simulink model "SetBelt"  (R2024a)
settings: Solver=FixedStepAuto  StartTime=0.0  StopTime=30  RelTol=1e-3
undefined symbols (not defined in the file): Dem_EventStatusType, enState_IgnitionKey
libraries: simulink x7, autosarlibnvm x3, autosarlibdem x2, dspswit3 x1
settings Model: Creator=buiqu  LastModifiedBy=buiqu
settings OptimizationCC: DefaultParameterBehavior=Inlined  EnhancedBackFolding=on  PassReuseOutputArgsAs=Individual arguments  ZeroExternalMemoryAtStartup=off  ZeroInternalMemoryAtStartup=off  OptimizeBlockOrder=speed  DifferentSizesBufferReuse=on  OptimizationCustomize=off  EfficientTunableParamExpr=on
settings DebuggingCC: ParameterTunabilityLossMsg=error
settings SFSimCC: MATLABDynamicMemAlloc=off
settings RTWCC: Description=AUTOSAR  SystemTargetFile=autosar.tlc  GenCodeOnly=on  TemplateMakefile=ert_default_tmf  DataTypeReplacement=CDataTypesFixedWidth
settings CodeAppCC: ForceParamTrailComments=on  IgnoreCustomStorageClasses=off  OperatorAnnotations=on  SimulinkDataObjDesc=on  SFDataObjDesc=on  InsertBlockDesc=on
settings STFCustomTargetCC: MultiwordLength=256  ParMdlRefBuildCompliant=on  CompOptLevelCompliant=on  CombineOutputUpdateFcns=on  SuppressErrorStatus=on  ERTCustomFileBanners=on  SupportNonFinite=off  SupportComplex=off  SupportContinuousTime=off  SupportNonInlinedSFcns=off  RemoveResetFunc=on  MATLABClassNameForMDSCustomization=Simulink.SoftwareTarget.ERTCustomization  AutosarCompliant=on  GRTInterface=off  LookupTableObjectStructAxisOrder=2,1,3,4,...  LUTObjectStructOrderEvenSpacing=Size,Table,Breakpoints  SystemTargetFile=autosar.tlc
settings ERTTargetCC: TargetLangStandard=C99 (ISO)  ConcurrentExecutionCompliant=off  SuppressErrorStatus=on  SupportNonFinite=off  SupportComplex=off  ModelStepFunctionPrototypeControlCompliant=off  CPPClassGenCompliant=off  AutosarCompliant=on  LookupTableObjectStructAxisOrder=2,1,3,4,...  LUTObjectStructOrderEvenSpacing=Size,Table,Breakpoints  InlinedParameterPlacement=NonHierarchical  ERTCustomFileTemplate=example_file_process.tlc  BooleanTrueId=TRUE  BooleanFalseId=FALSE

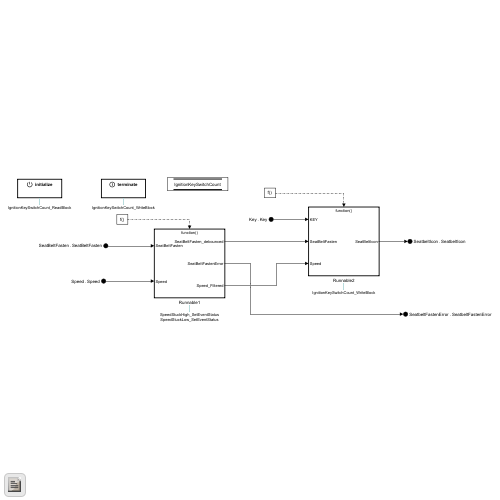
[thumbnail: Simulink's stored preview of the top-level diagram]
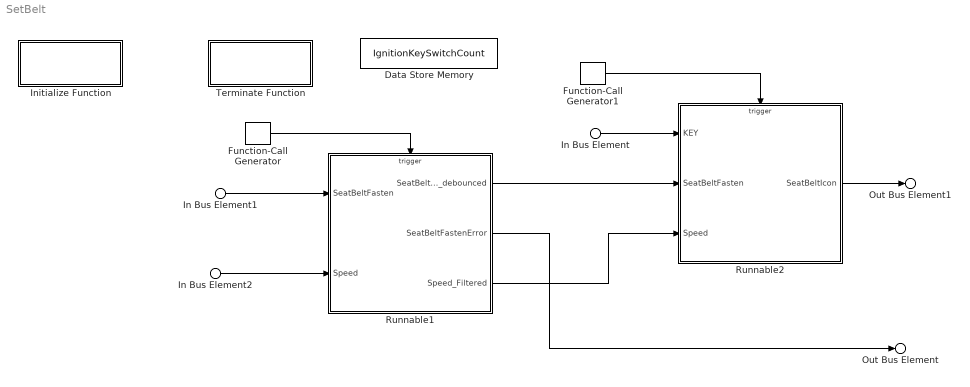
== system SetBelt ==
  In Bus Element : Inport  PortName=Key  Element=Key
  In Bus Element1 : Inport  Port=2  PortName=SeatBeltFasten  Element=SeatBeltFasten
  In Bus Element2 : Inport  Port=3  PortName=Speed  Element=Speed
  Data Store Memory : DataStoreMemory  DataStoreName=IgnitionKeySwitchCount  WriteAfterWriteMsg=warning  ShowAdditionalParam=off
  Function-Call Generator : simulink/Ports & Subsystems/Function-Call Generator  sample_time=1  numberOfIterations=1  DisallowWideOutput=off
  Function-Call Generator1 : simulink/Ports & Subsystems/Function-Call Generator  sample_time=1  numberOfIterations=1  DisallowWideOutput=off
  Initialize Function : Subsystem  TreatAsAtomicUnit=on
  Runnable1 : Subsystem  TreatAsAtomicUnit=on
  Runnable2 : Subsystem  TreatAsAtomicUnit=on
  Terminate Function : Subsystem  TreatAsAtomicUnit=on
  Out Bus Element1 : Outport  PortName=SeatbeltIcon  Element=SeatbeltIcon
  Out Bus Element : Outport  Port=2  PortName=SeatbeltFastenError  Element=SeatbeltFastenError
  wires:
  Runnable1/3(Speed_Filtered) -> Runnable2/3(Speed)
  Function-Call Generator/1 -> Runnable1/Trigger
  Runnable1/1(SeatBeltFasten_debounced) -> Runnable2/2(SeatBeltFasten)
  Function-Call Generator1/1 -> Runnable2/Trigger
  In Bus Element/1 -> Runnable2/1(KEY)
  In Bus Element1/1 -> Runnable1/1(SeatBeltFasten)
  In Bus Element2/1 -> Runnable1/2(Speed)
  Runnable1/2(SeatBeltFastenError) -> Out Bus Element/1
  Runnable2/1(SeatBeltIcon) -> Out Bus Element1/1

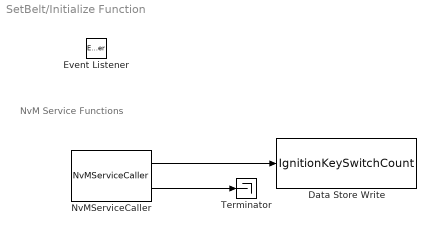
== system SetBelt/Initialize Function ==
  note: NvM Service Functions
  Data Store Write : DataStoreWrite  DataStoreName=IgnitionKeySwitchCount  IndexOptions=Index vector (dialog)  Indices=1  OutputSizes=1
  Event Listener : EventListener  DisableCoverage=on  EventName=reset
  NvMServiceCaller : autosarlibnvm/NvMServiceCaller  PortName=IgnitionKeySwitchCount  Operation=ReadBlock  ArgumentSpecification=uint8(1)  st=-1  ServiceImpl=autosar.bsw.NvMService  SyncToSchema=off
  Terminator : Terminator
  wires:
  NvMServiceCaller/2 -> Terminator/1
  NvMServiceCaller/1 -> Data Store Write/1

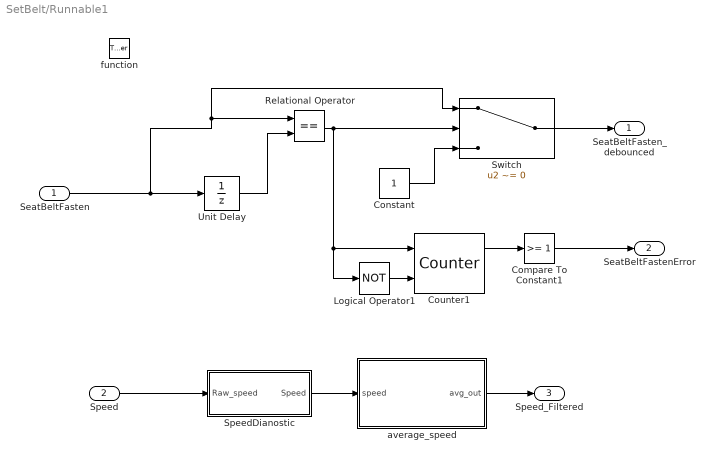
== system SetBelt/Runnable1 ==
  SeatBeltFasten : Inport
  Speed : Inport  Port=2  OutDataTypeStr=uint16
  function : TriggerPort  TriggerType=function-call  VariantControl=(inherit)
  Compare To Constant1 : simulink/Logic and Bit Operations/Compare To Constant  relop=>=  const=1  OutDataTypeStr=boolean
  Constant : Constant
  Counter1 : dspswit3/Counter  Direction=Up  CountEvent=Falling edge  CounterSize=User defined  MaxCount=3  InitialCount=0  Output=Count and Hit  HitValue=1  ResetInput=on  SamplesPerFrame=1  Ts=1  CntDtype=double  HitDtype=Boolean
  Logical Operator1 : Logic  Operator=NOT  AllPortsSameDT=off  OutDataTypeStr=boolean
  Relational Operator : RelationalOperator  Operator===  OutDataTypeStr=boolean  RndMeth=Simplest  InputSameDT=off
  SpeedDianostic : Subsystem
  Switch : Switch  Criteria=u2 ~= 0  OutDataTypeStr=boolean  SaturateOnIntegerOverflow=off  InputSameDT=off
  Unit Delay : UnitDelay  SampleTime=-1  HasFrameUpgradeWarning=on
  average_speed : MATLAB Function  TreatAsAtomicUnit=on
  SeatBeltFasten_debounced : Outport  OutMin=0  OutMax=1  OutDataTypeStr=boolean
  SeatBeltFastenError : Outport  Port=2  OutMin=0  OutMax=1  OutDataTypeStr=boolean
  Speed_Filtered : Outport  Port=3  OutDataTypeStr=uint16
  wires:
  SeatBeltFasten/1 -> Switch/1, Relational Operator/1, Unit Delay/1
  Speed/1 -> SpeedDianostic/1(Raw_speed)
  SpeedDianostic/1(Speed) -> average_speed/1(speed)
  average_speed/1(avg_out) -> Speed_Filtered/1
  Unit Delay/1 -> Relational Operator/2
  Relational Operator/1 -> Logical Operator1/1, Counter1/1, Switch/2
  Switch/1 -> SeatBeltFasten_debounced/1
  Constant/1 -> Switch/3
  Counter1/1 -> Compare To Constant1/1
  Compare To Constant1/1 -> SeatBeltFastenError/1
  Logical Operator1/1 -> Counter1/2

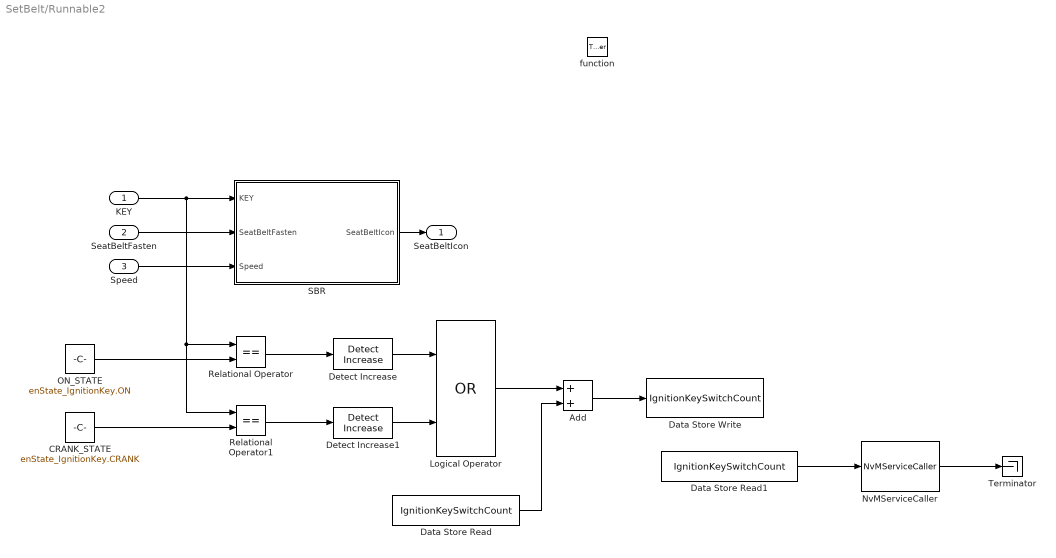
== system SetBelt/Runnable2 ==
  KEY : Inport  OutDataTypeStr=Enum: enState_IgnitionKey
  SeatBeltFasten : Inport  Port=2  OutDataTypeStr=boolean
  Speed : Inport  Port=3  OutDataTypeStr=uint16
  function : TriggerPort  TriggerType=function-call  VariantControl=(inherit)
  Add : Sum
  CRANK_STATE : Constant  Value=enState_IgnitionKey.CRANK  OutDataTypeStr=Enum: enState_IgnitionKey
  Data Store Read : DataStoreRead  DataStoreName=IgnitionKeySwitchCount  IndexOptions=Index vector (dialog)  Indices=1  OutputSizes=1
  Data Store Read1 : DataStoreRead  DataStoreName=IgnitionKeySwitchCount  IndexOptions=Index vector (dialog)  Indices=1  OutputSizes=1
  Data Store Write : DataStoreWrite  DataStoreName=IgnitionKeySwitchCount  IndexOptions=Index vector (dialog)  Indices=1  OutputSizes=1
  Detect Increase : simulink/Logic and Bit Operations/Detect Increase  vinit=0.0  OutDataTypeStr=boolean
  Detect Increase1 : simulink/Logic and Bit Operations/Detect Increase  vinit=0.0  OutDataTypeStr=boolean
  Logical Operator : Logic  Operator=OR  AllPortsSameDT=off  OutDataTypeStr=boolean
  NvMServiceCaller : autosarlibnvm/NvMServiceCaller  PortName=IgnitionKeySwitchCount  Operation=WriteBlock  ArgumentSpecification=uint8(1)  st=-1  ServiceImpl=autosar.bsw.NvMService  SyncToSchema=off
  ON_STATE : Constant  Value=enState_IgnitionKey.ON  OutDataTypeStr=Enum: enState_IgnitionKey
  Relational Operator : RelationalOperator  Operator===  OutDataTypeStr=boolean  RndMeth=Simplest  InputSameDT=off
  Relational Operator1 : RelationalOperator  Operator===  OutDataTypeStr=boolean  RndMeth=Simplest  InputSameDT=off
  SBR : Subsystem
  Terminator : Terminator
  SeatBeltIcon : Outport  OutDataTypeStr=boolean
  wires:
  KEY/1 -> Relational Operator1/1, Relational Operator/1, SBR/1(KEY)
  SeatBeltFasten/1 -> SBR/2(SeatBeltFasten)
  Speed/1 -> SBR/3(Speed)
  ON_STATE/1 -> Relational Operator/2
  CRANK_STATE/1 -> Relational Operator1/2
  Relational Operator/1 -> Detect Increase/1
  Relational Operator1/1 -> Detect Increase1/1
  Detect Increase1/1 -> Logical Operator/2
  Detect Increase/1 -> Logical Operator/1
  Logical Operator/1 -> Add/1
  Data Store Read/1 -> Add/2
  Add/1 -> Data Store Write/1
  Data Store Read1/1 -> NvMServiceCaller/1
  NvMServiceCaller/1 -> Terminator/1
  SBR/1(SeatBeltIcon) -> SeatBeltIcon/1

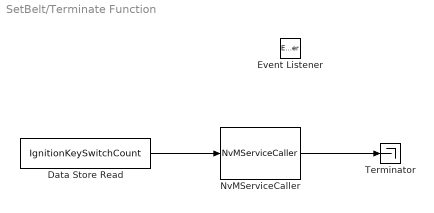
== system SetBelt/Terminate Function ==
  Data Store Read : DataStoreRead  DataStoreName=IgnitionKeySwitchCount  IndexOptions=Index vector (dialog)  Indices=1  OutputSizes=1
  Event Listener : EventListener  DisableCoverage=on  EventType=Terminate  EventName=reset
  NvMServiceCaller : autosarlibnvm/NvMServiceCaller  PortName=IgnitionKeySwitchCount  Operation=WriteBlock  ArgumentSpecification=uint8(1)  st=-1  ServiceImpl=autosar.bsw.NvMService  SyncToSchema=off
  Terminator : Terminator
  wires:
  Data Store Read/1 -> NvMServiceCaller/1
  NvMServiceCaller/1 -> Terminator/1

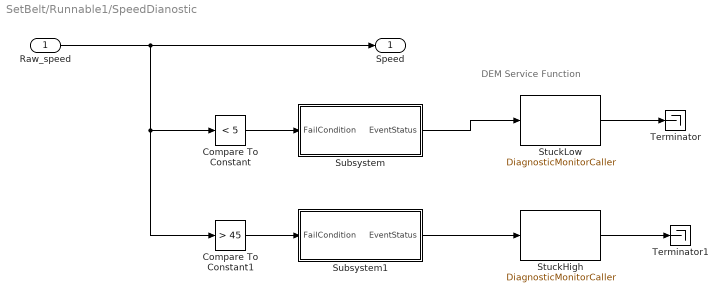
== system SetBelt/Runnable1/SpeedDianostic ==
  note: DEM Service Function
  Raw_speed : Inport  OutDataTypeStr=uint16
  Compare To Constant : simulink/Logic and Bit Operations/Compare To Constant  relop=<  const=5  OutDataTypeStr=boolean
  Compare To Constant1 : simulink/Logic and Bit Operations/Compare To Constant  relop=>  const=45  OutDataTypeStr=boolean
  StuckHigh : autosarlibdem/DiagnosticMonitorCaller  PortName=SpeedStuckHigh  Operation=SetEventStatus  Datatype=Enum: Dem_EventStatusType  st=-1  ServiceImpl=autosar.bsw.DemDiagnosticMonitor  SyncToSchema=off
  StuckLow : autosarlibdem/DiagnosticMonitorCaller  PortName=SpeedStuckLow  Operation=SetEventStatus  Datatype=Enum: Dem_EventStatusType  st=-1  ServiceImpl=autosar.bsw.DemDiagnosticMonitor  SyncToSchema=off
  Subsystem : Subsystem
  Subsystem1 : Subsystem
  Terminator : Terminator
  Terminator1 : Terminator
  Speed : Outport
  wires:
  Raw_speed/1 -> Compare To Constant1/1, Compare To Constant/1, Speed/1
  Compare To Constant/1 -> Subsystem/1(FailCondition)
  Compare To Constant1/1 -> Subsystem1/1(FailCondition)
  Subsystem1/1(EventStatus) -> StuckHigh/1
  Subsystem/1(EventStatus) -> StuckLow/1
  StuckHigh/1 -> Terminator1/1
  StuckLow/1 -> Terminator/1

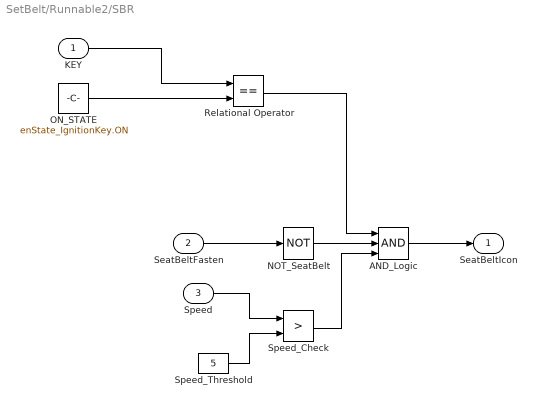
== system SetBelt/Runnable2/SBR ==
  KEY : Inport  OutDataTypeStr=Enum: enState_IgnitionKey
  SeatBeltFasten : Inport  Port=2  OutDataTypeStr=boolean
  Speed : Inport  Port=3  OutDataTypeStr=uint16
  AND_Logic : Logic  Inputs=3  AllPortsSameDT=off  OutDataTypeStr=boolean
  NOT_SeatBelt : Logic  Operator=NOT  AllPortsSameDT=off  OutDataTypeStr=boolean
  ON_STATE : Constant  Value=enState_IgnitionKey.ON  OutDataTypeStr=Enum: enState_IgnitionKey
  Relational Operator : RelationalOperator  Operator===  OutDataTypeStr=boolean  RndMeth=Simplest  InputSameDT=off
  Speed_Check : RelationalOperator  Operator=>  OutDataTypeStr=boolean  RndMeth=Simplest  InputSameDT=off
  Speed_Threshold : Constant  Value=5
  SeatBeltIcon : Outport  OutDataTypeStr=boolean
  wires:
  SeatBeltFasten/1 -> NOT_SeatBelt/1
  Speed/1 -> Speed_Check/1
  Speed_Threshold/1 -> Speed_Check/2
  NOT_SeatBelt/1 -> AND_Logic/2
  Speed_Check/1 -> AND_Logic/3
  AND_Logic/1 -> SeatBeltIcon/1
  ON_STATE/1 -> Relational Operator/2
  Relational Operator/1 -> AND_Logic/1
  KEY/1 -> Relational Operator/1

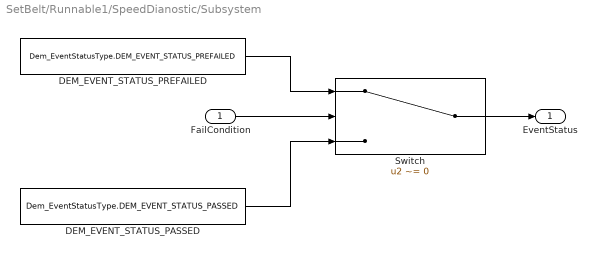
== system SetBelt/Runnable1/SpeedDianostic/Subsystem ==
  FailCondition : Inport  OutDataTypeStr=boolean
  DEM_EVENT_STATUS_PASSED : Constant  Value=Dem_EventStatusType.DEM_EVENT_STATUS_PASSED  OutDataTypeStr=Enum: Dem_EventStatusType
  DEM_EVENT_STATUS_PREFAILED : Constant  Value=Dem_EventStatusType.DEM_EVENT_STATUS_PREFAILED  OutDataTypeStr=Enum: Dem_EventStatusType
  Switch : Switch  Criteria=u2 ~= 0  OutDataTypeStr=Enum: Dem_EventStatusType  SaturateOnIntegerOverflow=off  InputSameDT=off
  EventStatus : Outport  OutDataTypeStr=Enum: Dem_EventStatusType
  wires:
  Switch/1 -> EventStatus/1
  FailCondition/1 -> Switch/2
  DEM_EVENT_STATUS_PREFAILED/1 -> Switch/1
  DEM_EVENT_STATUS_PASSED/1 -> Switch/3

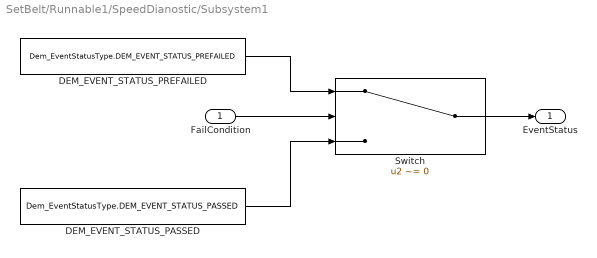
== system SetBelt/Runnable1/SpeedDianostic/Subsystem1 ==
  FailCondition : Inport  OutDataTypeStr=boolean
  DEM_EVENT_STATUS_PASSED : Constant  Value=Dem_EventStatusType.DEM_EVENT_STATUS_PASSED  OutDataTypeStr=Enum: Dem_EventStatusType
  DEM_EVENT_STATUS_PREFAILED : Constant  Value=Dem_EventStatusType.DEM_EVENT_STATUS_PREFAILED  OutDataTypeStr=Enum: Dem_EventStatusType
  Switch : Switch  Criteria=u2 ~= 0  OutDataTypeStr=Enum: Dem_EventStatusType  SaturateOnIntegerOverflow=off  InputSameDT=off
  EventStatus : Outport  OutDataTypeStr=Enum: Dem_EventStatusType
  wires:
  Switch/1 -> EventStatus/1
  FailCondition/1 -> Switch/2
  DEM_EVENT_STATUS_PREFAILED/1 -> Switch/1
  DEM_EVENT_STATUS_PASSED/1 -> Switch/3

== matlab function SetBelt/Runnable1/average_speed ==
  data: speed input; avg_out output
function avg_out = runningAverage(speed)
%#codegen

    persistent buffer index count

    N = 5;  

    if isempty(buffer)
        buffer = zeros(1, N);  % Buffer 5 phần tử
        index = 1;             % Vị trí ghi đầu tiên
        count = 0;             % Số lượng phần tử đã ghi
    end

    buffer(index) = double(speed);
    index = mod(index, N) + 1;
    count = min(count + 1, N);

    % Tính trung bình
    avg_out = uint16(sum(buffer) / count);
end
